simulink model "Week11_Simulation_Control"  (R2017b)
settings: Solver=ode4  StartTime=0.0  StopTime=20  FixedStep=1e-3  RelTol=1e-3  EnableMultiTasking=on
values from neighbouring files (symbols this model uses):
  g = 9.8    [Parameters.m]
  l1 = 3    [Parameters.m]
  l2 = 2    [Parameters.m]
  m1 = 3    [Parameters.m]
  m2 = 2    [Parameters.m]
undefined symbols (not defined in the file or in its folder): DiscIntNeverNeededParam
libraries: simulink x16, dspinverses x6
(part 2 of 2)

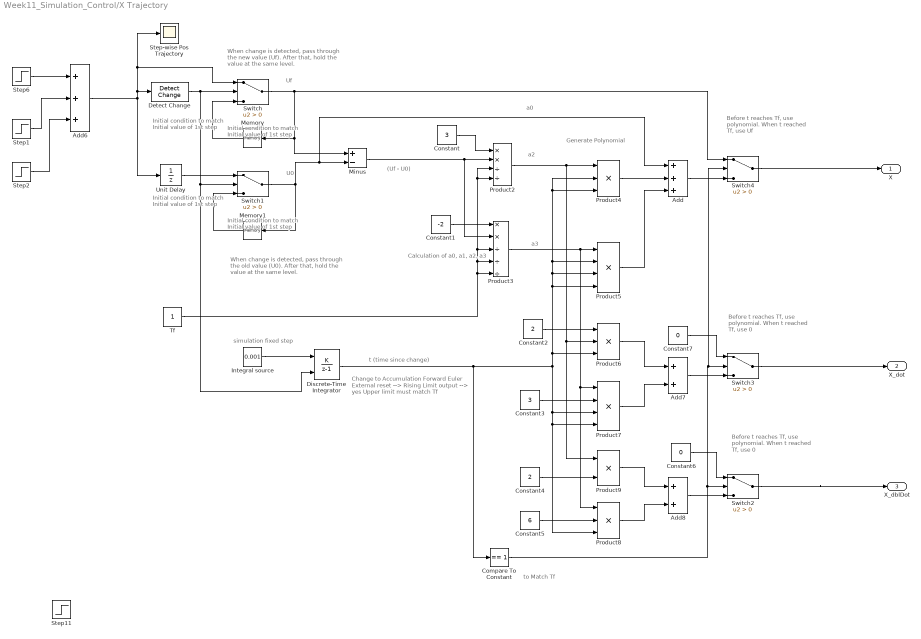
== system Week11_Simulation_Control/X Trajectory ==
  note: Initial condition
      | to match
      | Initial value
      | of 1st step
  note: Generate Polynomial
  note: Calculation of
      | a0, a1, a2, a3
  note: Before t reaches Tf,
      | use polynomial.
      | When t reached Tf,
      | use Uf
  note: to Match Tf
  note: t (time since change)
  note: When change is detected, pass through
      | the old value (U0). After that, hold the
      | value at the same level.
  note: simulation fixed step
  note: Change to Accumulation Forward Euler
      | External reset --> Rising
      | Limit output --> yes
      | Upper limit must match Tf
  note: a3
  note: a2
  note: Uf
  note: U0
  note: When change is detected, pass through
      | the new value (Uf). After that, hold the
      | value at the same level.
  note: Before t reaches Tf,
      | use polynomial.
      | When t reached Tf,
      | use 0
  note: Before t reaches Tf,
      | use polynomial.
      | When t reached Tf,
      | use 0
  note: (Uf - U0)
  note: a0
  note: Initial condition
      | to match
      | Initial value
      | of 1st step
  note: Initial condition
      | to match
      | Initial value
      | of 1st step
  note: Initial condition
      | to match
      | Initial value
      | of 1st step
  Add : Sum  Inputs=3
  Add6 : Sum  Inputs=3
  Add7 : Sum  Inputs=2
  Add8 : Sum  Inputs=2
  Compare To Constant : simulink/Logic and Bit Operations/Compare To Constant  relop===  const=1  OutDataTypeStr=boolean
  Constant : Constant  Value=3
  Constant1 : Constant  Value=-2
  Constant2 : Constant  Value=2
  Constant3 : Constant  Value=3
  Constant4 : Constant  Value=2
  Constant5 : Constant  Value=6
  Constant6 : Constant  Value=0
  Constant7 : Constant  Value=0
  Detect Change : simulink/Logic and Bit Operations/Detect Change  vinit=5  InputProcessing=Inherited  OutDataTypeStr=boolean
  Discrete-Time Integrator : DiscreteIntegrator  IntegratorMethod=Accumulation: Forward Euler  gainval=1  ExternalReset=rising  InitialConditionSetting=State (most efficient)  SampleTime=-1  LimitOutput=on  UpperSaturationLimit=1  ICPrevOutput=DiscIntNeverNeededParam  ICPrevScaledInput=DiscIntNeverNeededParam
  Integral source : Constant  Value=0.001
  Memory : Memory  InitialCondition=5  InheritSampleTime=on
  Memory1 : Memory  InitialCondition=5  InheritSampleTime=on
  Minus : Sum  Inputs=+-
  Product2 : Product  Inputs=**//
  Product3 : Product  Inputs=**///
  Product4 : Product  Inputs=3
  Product5 : Product  Inputs=4
  Product6 : Product  Inputs=3
  Product7 : Product  Inputs=4
  Product8 : Product  Inputs=3
  Product9 : Product
  Step-wise Pos Trajectory : Scope
  Step1 : Step  Time=9  After=-6  SampleTime=0
  Step11 : Step  Time=17  After=-2  SampleTime=0
  Step2 : Step  Time=15  After=6  SampleTime=0
  Step6 : Step  Time=3  Before=5  After=3  SampleTime=0
  Switch{,1..4} (5 alike) : Switch  Criteria=u2 > Threshold
  Tf : Constant
  Unit Delay : UnitDelay  InitialCondition=5  SampleTime=-1
  X : Outport
  X_dot : Outport  Port=2
  X_dblDot : Outport  Port=3
  wires:
  Add8/1 -> Switch2/3
  Product9/1 -> Add8/1
  Constant7/1 -> Switch3/1
  Constant/1 -> Product2/1
  Integral source/1 -> Discrete-Time Integrator/1
  Add/1 -> Switch4/3
  Product4/1 -> Add/2
  Switch3/1 -> X_dot/1
  Compare To Constant/1 -> Switch4/2, Switch3/2, Switch2/2
  Switch2/1 -> X_dblDot/1
  Constant6/1 -> Switch2/1
  Constant4/1 -> Product9/2
  Product8/1 -> Add8/2
  Constant5/1 -> Product8/2
  Product5/1 -> Add/3
  Product7/1 -> Add7/2
  Constant3/1 -> Product7/2
  Detect Change/1 -> Discrete-Time Integrator/2, Switch1/2, Switch/2
  Discrete-Time Integrator/1 -> Compare To Constant/1, Product7/3, Product8/3, Product7/4, Product6/3, Product5/4, Product5/3, Product5/2, Product4/3, Product4/2
  Product3/1 -> Product8/1, Product7/1, Product5/1
  Constant1/1 -> Product3/1
  Product6/1 -> Add7/1
  Tf/1 -> Product3/5, Product3/4, Product3/3, Product2/4, Product2/3
  Add7/1 -> Switch3/3
  Minus/1 -> Product3/2, Product2/2
  Unit Delay/1 -> Switch1/1
  Memory1/1 -> Switch1/3
  Switch1/1 -> Memory1/1, Add/1, Minus/2
  Constant2/1 -> Product6/1
  Product2/1 -> Product9/1, Product6/2, Product4/1
  Memory/1 -> Switch/3
  Switch/1 -> Minus/1, Memory/1, Switch4/1
  Step6/1 -> Add6/1
  Step1/1 -> Add6/2
  Step2/1 -> Add6/3
  Add6/1 -> Unit Delay/1, Detect Change/1, Step-wise Pos Trajectory/1, Switch/1
  Switch4/1 -> X/1

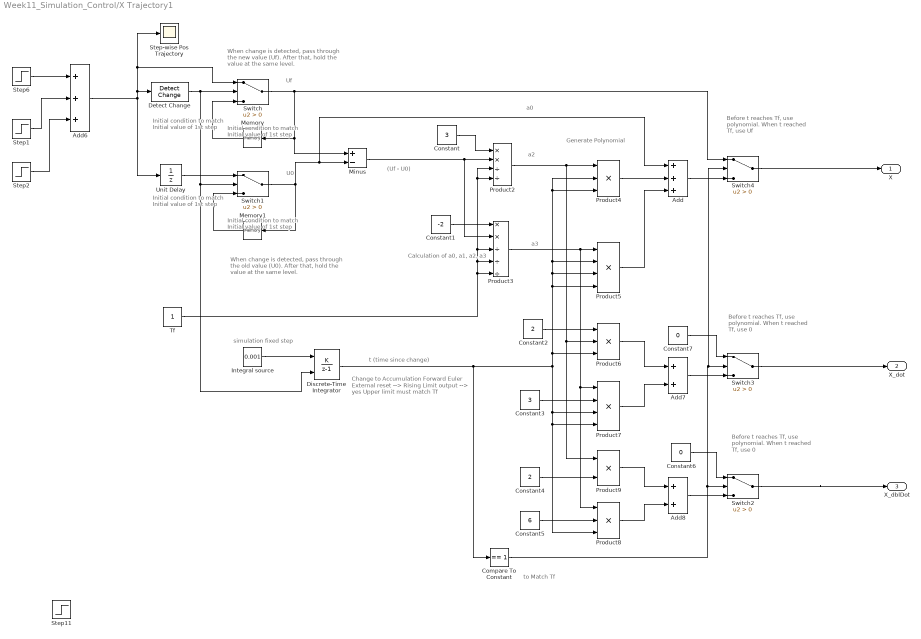
== system Week11_Simulation_Control/X Trajectory1 ==
  note: Initial condition
      | to match
      | Initial value
      | of 1st step
  note: Generate Polynomial
  note: Calculation of
      | a0, a1, a2, a3
  note: Before t reaches Tf,
      | use polynomial.
      | When t reached Tf,
      | use Uf
  note: to Match Tf
  note: t (time since change)
  note: When change is detected, pass through
      | the old value (U0). After that, hold the
      | value at the same level.
  note: simulation fixed step
  note: Change to Accumulation Forward Euler
      | External reset --> Rising
      | Limit output --> yes
      | Upper limit must match Tf
  note: a3
  note: a2
  note: Uf
  note: U0
  note: When change is detected, pass through
      | the new value (Uf). After that, hold the
      | value at the same level.
  note: Before t reaches Tf,
      | use polynomial.
      | When t reached Tf,
      | use 0
  note: Before t reaches Tf,
      | use polynomial.
      | When t reached Tf,
      | use 0
  note: (Uf - U0)
  note: a0
  note: Initial condition
      | to match
      | Initial value
      | of 1st step
  note: Initial condition
      | to match
      | Initial value
      | of 1st step
  note: Initial condition
      | to match
      | Initial value
      | of 1st step
  Add : Sum  Inputs=3
  Add6 : Sum  Inputs=3
  Add7 : Sum  Inputs=2
  Add8 : Sum  Inputs=2
  Compare To Constant : simulink/Logic and Bit Operations/Compare To Constant  relop===  const=1  OutDataTypeStr=boolean
  Constant : Constant  Value=3
  Constant1 : Constant  Value=-2
  Constant2 : Constant  Value=2
  Constant3 : Constant  Value=3
  Constant4 : Constant  Value=2
  Constant5 : Constant  Value=6
  Constant6 : Constant  Value=0
  Constant7 : Constant  Value=0
  Detect Change : simulink/Logic and Bit Operations/Detect Change  vinit=5  InputProcessing=Inherited  OutDataTypeStr=boolean
  Discrete-Time Integrator : DiscreteIntegrator  IntegratorMethod=Accumulation: Forward Euler  gainval=1  ExternalReset=rising  InitialConditionSetting=State (most efficient)  SampleTime=-1  LimitOutput=on  UpperSaturationLimit=1  ICPrevOutput=DiscIntNeverNeededParam  ICPrevScaledInput=DiscIntNeverNeededParam
  Integral source : Constant  Value=0.001
  Memory : Memory  InitialCondition=5  InheritSampleTime=on
  Memory1 : Memory  InitialCondition=5  InheritSampleTime=on
  Minus : Sum  Inputs=+-
  Product2 : Product  Inputs=**//
  Product3 : Product  Inputs=**///
  Product4 : Product  Inputs=3
  Product5 : Product  Inputs=4
  Product6 : Product  Inputs=3
  Product7 : Product  Inputs=4
  Product8 : Product  Inputs=3
  Product9 : Product
  Step-wise Pos Trajectory : Scope
  Step1 : Step  Time=9  After=-6  SampleTime=0
  Step11 : Step  Time=17  After=-2  SampleTime=0
  Step2 : Step  Time=15  After=6  SampleTime=0
  Step6 : Step  Time=3  Before=5  After=3  SampleTime=0
  Switch{,1..4} (5 alike) : Switch  Criteria=u2 > Threshold
  Tf : Constant
  Unit Delay : UnitDelay  InitialCondition=5  SampleTime=-1
  X : Outport
  X_dot : Outport  Port=2
  X_dblDot : Outport  Port=3
  wires:
  Add8/1 -> Switch2/3
  Product9/1 -> Add8/1
  Constant7/1 -> Switch3/1
  Constant/1 -> Product2/1
  Integral source/1 -> Discrete-Time Integrator/1
  Add/1 -> Switch4/3
  Product4/1 -> Add/2
  Switch3/1 -> X_dot/1
  Compare To Constant/1 -> Switch4/2, Switch3/2, Switch2/2
  Switch2/1 -> X_dblDot/1
  Constant6/1 -> Switch2/1
  Constant4/1 -> Product9/2
  Product8/1 -> Add8/2
  Constant5/1 -> Product8/2
  Product5/1 -> Add/3
  Product7/1 -> Add7/2
  Constant3/1 -> Product7/2
  Detect Change/1 -> Discrete-Time Integrator/2, Switch1/2, Switch/2
  Discrete-Time Integrator/1 -> Compare To Constant/1, Product7/3, Product8/3, Product7/4, Product6/3, Product5/4, Product5/3, Product5/2, Product4/3, Product4/2
  Product3/1 -> Product8/1, Product7/1, Product5/1
  Constant1/1 -> Product3/1
  Product6/1 -> Add7/1
  Tf/1 -> Product3/5, Product3/4, Product3/3, Product2/4, Product2/3
  Add7/1 -> Switch3/3
  Minus/1 -> Product3/2, Product2/2
  Unit Delay/1 -> Switch1/1
  Memory1/1 -> Switch1/3
  Switch1/1 -> Memory1/1, Add/1, Minus/2
  Constant2/1 -> Product6/1
  Product2/1 -> Product9/1, Product6/2, Product4/1
  Memory/1 -> Switch/3
  Switch/1 -> Minus/1, Memory/1, Switch4/1
  Step6/1 -> Add6/1
  Step1/1 -> Add6/2
  Step2/1 -> Add6/3
  Add6/1 -> Unit Delay/1, Detect Change/1, Step-wise Pos Trajectory/1, Switch/1
  Switch4/1 -> X/1

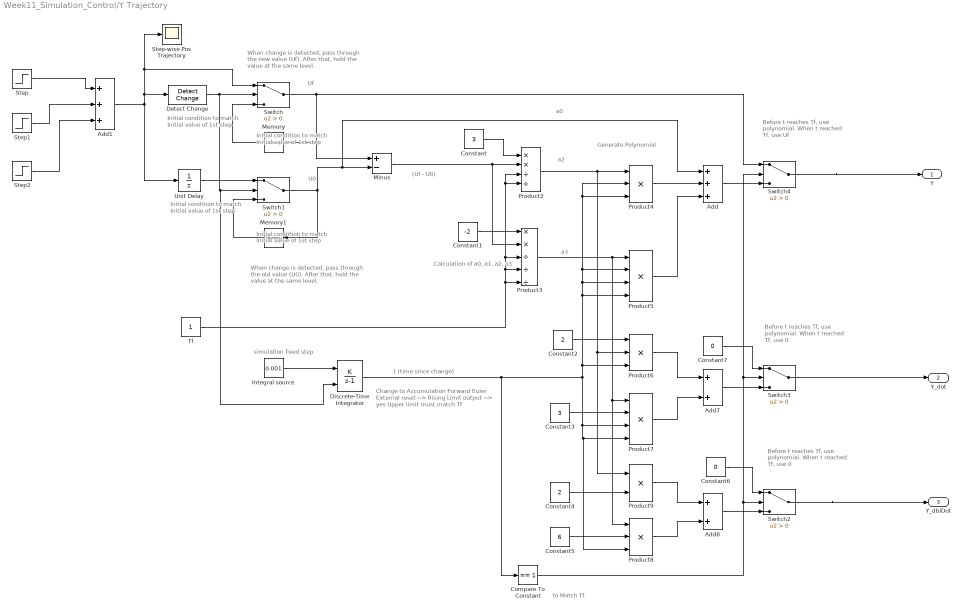
== system Week11_Simulation_Control/Y Trajectory ==
  note: a0
  note: (Uf - U0)
  note: Before t reaches Tf,
      | use polynomial.
      | When t reached Tf,
      | use 0
  note: Before t reaches Tf,
      | use polynomial.
      | When t reached Tf,
      | use 0
  note: When change is detected, pass through
      | the new value (Uf). After that, hold the
      | value at the same level.
  note: U0
  note: Uf
  note: a2
  note: a3
  note: Change to Accumulation Forward Euler
      | External reset --> Rising
      | Limit output --> yes
      | Upper limit must match Tf
  note: simulation fixed step
  note: When change is detected, pass through
      | the old value (U0). After that, hold the
      | value at the same level.
  note: t (time since change)
  note: to Match Tf
  note: Before t reaches Tf,
      | use polynomial.
      | When t reached Tf,
      | use Uf
  note: Calculation of
      | a0, a1, a2, a3
  note: Generate Polynomial
  note: Initial condition
      | to match
      | Initial value
      | of 1st step
  note: Initial condition
      | to match
      | Initial value
      | of 1st step
  note: Initial condition
      | to match
      | Initial value
      | of 1st step
  note: Initial condition
      | to match
      | Initial value
      | of 1st step
  Add : Sum  Inputs=3
  Add1 : Sum  Inputs=3
  Add7 : Sum  Inputs=2
  Add8 : Sum  Inputs=2
  Compare To Constant : simulink/Logic and Bit Operations/Compare To Constant  relop===  const=1  OutDataTypeStr=boolean
  Constant : Constant  Value=3
  Constant1 : Constant  Value=-2
  Constant2 : Constant  Value=2
  Constant3 : Constant  Value=3
  Constant4 : Constant  Value=2
  Constant5 : Constant  Value=6
  Constant6 : Constant  Value=0
  Constant7 : Constant  Value=0
  Detect Change : simulink/Logic and Bit Operations/Detect Change  vinit=0  InputProcessing=Inherited  OutDataTypeStr=boolean
  Discrete-Time Integrator : DiscreteIntegrator  IntegratorMethod=Accumulation: Forward Euler  gainval=1  ExternalReset=rising  InitialConditionSetting=State (most efficient)  SampleTime=-1  LimitOutput=on  UpperSaturationLimit=1  ICPrevOutput=DiscIntNeverNeededParam  ICPrevScaledInput=DiscIntNeverNeededParam
  Integral source : Constant  Value=0.001
  Memory : Memory  InheritSampleTime=on
  Memory1 : Memory  InheritSampleTime=on
  Minus : Sum  Inputs=+-
  Product2 : Product  Inputs=**//
  Product3 : Product  Inputs=**///
  Product4 : Product  Inputs=3
  Product5 : Product  Inputs=4
  Product6 : Product  Inputs=3
  Product7 : Product  Inputs=4
  Product8 : Product  Inputs=3
  Product9 : Product
  Step : Step  Time=6  After=3.5  SampleTime=0
  Step-wise Pos Trajectory : Scope
  Step1 : Step  Time=12  After=-2  SampleTime=0
  Step2 : Step  Time=18  After=-2  SampleTime=0
  Switch{,1..4} (5 alike) : Switch  Criteria=u2 > Threshold
  Tf : Constant
  Unit Delay : UnitDelay  SampleTime=-1
  Y : Outport
  Y_dot : Outport  Port=2
  Y_dblDot : Outport  Port=3
  wires:
  Switch/1 -> Switch4/1, Memory/1, Minus/1
  Memory/1 -> Switch/3
  Product2/1 -> Product4/1, Product6/2, Product9/1
  Constant2/1 -> Product6/1
  Switch1/1 -> Minus/2, Add/1, Memory1/1
  Memory1/1 -> Switch1/3
  Unit Delay/1 -> Switch1/1
  Minus/1 -> Product2/2, Product3/2
  Add7/1 -> Switch3/3
  Tf/1 -> Product2/3, Product2/4, Product3/3, Product3/4, Product3/5
  Product6/1 -> Add7/1
  Constant1/1 -> Product3/1
  Product3/1 -> Product5/1, Product7/1, Product8/1
  Discrete-Time Integrator/1 -> Product4/2, Product4/3, Product5/2, Product5/3, Product5/4, Product6/3, Product7/4, Product8/3, Product7/3, Compare To Constant/1
  Detect Change/1 -> Switch/2, Switch1/2, Discrete-Time Integrator/2
  Constant3/1 -> Product7/2
  Product7/1 -> Add7/2
  Product5/1 -> Add/3
  Constant5/1 -> Product8/2
  Product8/1 -> Add8/2
  Constant4/1 -> Product9/2
  Constant6/1 -> Switch2/1
  Switch2/1 -> Y_dblDot/1
  Compare To Constant/1 -> Switch2/2, Switch3/2, Switch4/2
  Switch3/1 -> Y_dot/1
  Product4/1 -> Add/2
  Add1/1 -> Unit Delay/1, Detect Change/1, Step-wise Pos Trajectory/1, Switch/1
  Add/1 -> Switch4/3
  Switch4/1 -> Y/1
  Integral source/1 -> Discrete-Time Integrator/1
  Constant/1 -> Product2/1
  Constant7/1 -> Switch3/1
  Product9/1 -> Add8/1
  Add8/1 -> Switch2/3
  Step1/1 -> Add1/2
  Step/1 -> Add1/1
  Step2/1 -> Add1/3

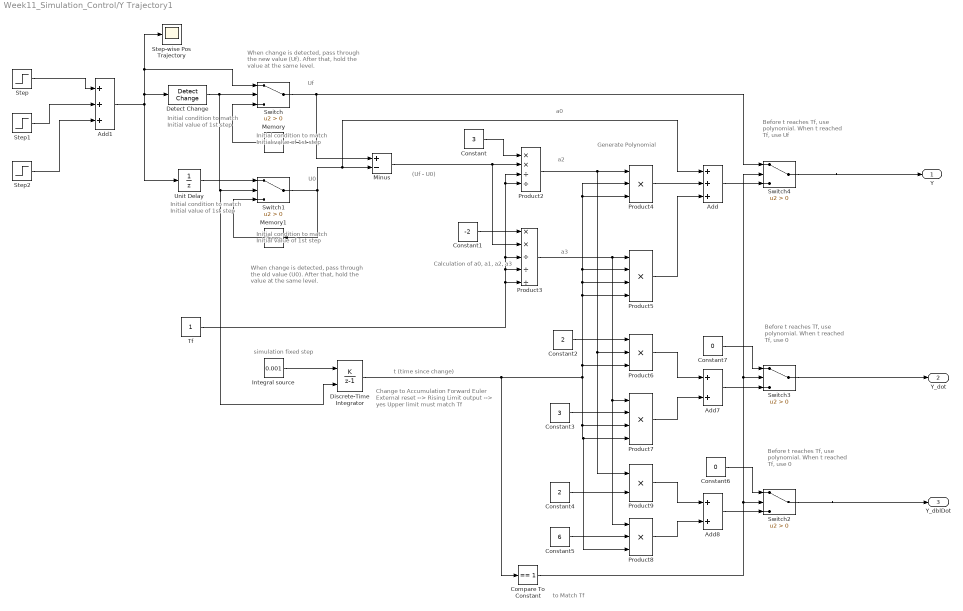
== system Week11_Simulation_Control/Y Trajectory1 ==
  note: a0
  note: (Uf - U0)
  note: Before t reaches Tf,
      | use polynomial.
      | When t reached Tf,
      | use 0
  note: Before t reaches Tf,
      | use polynomial.
      | When t reached Tf,
      | use 0
  note: When change is detected, pass through
      | the new value (Uf). After that, hold the
      | value at the same level.
  note: U0
  note: Uf
  note: a2
  note: a3
  note: Change to Accumulation Forward Euler
      | External reset --> Rising
      | Limit output --> yes
      | Upper limit must match Tf
  note: simulation fixed step
  note: When change is detected, pass through
      | the old value (U0). After that, hold the
      | value at the same level.
  note: t (time since change)
  note: to Match Tf
  note: Before t reaches Tf,
      | use polynomial.
      | When t reached Tf,
      | use Uf
  note: Calculation of
      | a0, a1, a2, a3
  note: Generate Polynomial
  note: Initial condition
      | to match
      | Initial value
      | of 1st step
  note: Initial condition
      | to match
      | Initial value
      | of 1st step
  note: Initial condition
      | to match
      | Initial value
      | of 1st step
  note: Initial condition
      | to match
      | Initial value
      | of 1st step
  Add : Sum  Inputs=3
  Add1 : Sum  Inputs=3
  Add7 : Sum  Inputs=2
  Add8 : Sum  Inputs=2
  Compare To Constant : simulink/Logic and Bit Operations/Compare To Constant  relop===  const=1  OutDataTypeStr=boolean
  Constant : Constant  Value=3
  Constant1 : Constant  Value=-2
  Constant2 : Constant  Value=2
  Constant3 : Constant  Value=3
  Constant4 : Constant  Value=2
  Constant5 : Constant  Value=6
  Constant6 : Constant  Value=0
  Constant7 : Constant  Value=0
  Detect Change : simulink/Logic and Bit Operations/Detect Change  vinit=0  InputProcessing=Inherited  OutDataTypeStr=boolean
  Discrete-Time Integrator : DiscreteIntegrator  IntegratorMethod=Accumulation: Forward Euler  gainval=1  ExternalReset=rising  InitialConditionSetting=State (most efficient)  SampleTime=-1  LimitOutput=on  UpperSaturationLimit=1  ICPrevOutput=DiscIntNeverNeededParam  ICPrevScaledInput=DiscIntNeverNeededParam
  Integral source : Constant  Value=0.001
  Memory : Memory  InheritSampleTime=on
  Memory1 : Memory  InheritSampleTime=on
  Minus : Sum  Inputs=+-
  Product2 : Product  Inputs=**//
  Product3 : Product  Inputs=**///
  Product4 : Product  Inputs=3
  Product5 : Product  Inputs=4
  Product6 : Product  Inputs=3
  Product7 : Product  Inputs=4
  Product8 : Product  Inputs=3
  Product9 : Product
  Step : Step  Time=6  After=3.5  SampleTime=0
  Step-wise Pos Trajectory : Scope
  Step1 : Step  Time=12  After=-2  SampleTime=0
  Step2 : Step  Time=18  After=-2  SampleTime=0
  Switch{,1..4} (5 alike) : Switch  Criteria=u2 > Threshold
  Tf : Constant
  Unit Delay : UnitDelay  SampleTime=-1
  Y : Outport
  Y_dot : Outport  Port=2
  Y_dblDot : Outport  Port=3
  wires:
  Switch/1 -> Switch4/1, Memory/1, Minus/1
  Memory/1 -> Switch/3
  Product2/1 -> Product4/1, Product6/2, Product9/1
  Constant2/1 -> Product6/1
  Switch1/1 -> Minus/2, Add/1, Memory1/1
  Memory1/1 -> Switch1/3
  Unit Delay/1 -> Switch1/1
  Minus/1 -> Product2/2, Product3/2
  Add7/1 -> Switch3/3
  Tf/1 -> Product2/3, Product2/4, Product3/3, Product3/4, Product3/5
  Product6/1 -> Add7/1
  Constant1/1 -> Product3/1
  Product3/1 -> Product5/1, Product7/1, Product8/1
  Discrete-Time Integrator/1 -> Product4/2, Product4/3, Product5/2, Product5/3, Product5/4, Product6/3, Product7/4, Product8/3, Product7/3, Compare To Constant/1
  Detect Change/1 -> Switch/2, Switch1/2, Discrete-Time Integrator/2
  Constant3/1 -> Product7/2
  Product7/1 -> Add7/2
  Product5/1 -> Add/3
  Constant5/1 -> Product8/2
  Product8/1 -> Add8/2
  Constant4/1 -> Product9/2
  Constant6/1 -> Switch2/1
  Switch2/1 -> Y_dblDot/1
  Compare To Constant/1 -> Switch2/2, Switch3/2, Switch4/2
  Switch3/1 -> Y_dot/1
  Product4/1 -> Add/2
  Add1/1 -> Unit Delay/1, Detect Change/1, Step-wise Pos Trajectory/1, Switch/1
  Add/1 -> Switch4/3
  Switch4/1 -> Y/1
  Integral source/1 -> Discrete-Time Integrator/1
  Constant/1 -> Product2/1
  Constant7/1 -> Switch3/1
  Product9/1 -> Add8/1
  Add8/1 -> Switch2/3
  Step1/1 -> Add1/2
  Step/1 -> Add1/1
  Step2/1 -> Add1/3
